simulink model "Punto1"  (R2017b)
settings: Solver=VariableStepAuto  StartTime=0.0  StopTime=5  RelTol=1e-3
values from neighbouring files (symbols this model uses):
  dc = [.4 4.2 3]    [Practica5.m]    (also in punto1.m)
  ddc = ddc(2:end)    [Practica5.m]    (also in punto1.m = [1 -0.8251 -0.1748])
  nc = 1    [Practica5.m]    (also in punto1.m)
  ndc = [dd]    [Practica5.m]    (also in punto1.m = [9.4518 -6.5019 0.0491])
  T0 = .5    (= 0.5)    [Practica5.m]    (also in punto1.m = 0.02)
settings Model: Creator=Agustin  LastModifiedBy=Agustin

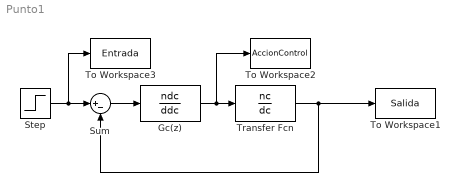
== system Punto1 ==
  Gc(z) : DiscreteTransferFcn  Numerator=ndc  Denominator=ddc  SampleTime=T0
  Step : Step  Time=0  SampleTime=T0
  Sum : Sum  Inputs=|+-
  To Workspace1 : ToWorkspace  VariableName=Salida  SaveFormat=Timeseries  SampleTime=-1
  To Workspace2 : ToWorkspace  VariableName=AccionControl  SaveFormat=Timeseries  SampleTime=-1
  To Workspace3 : ToWorkspace  VariableName=Entrada  SaveFormat=Timeseries  SampleTime=-1
  Transfer Fcn : TransferFcn  Numerator=nc  Denominator=dc
  wires:
  Transfer Fcn/1 -> To Workspace1/1, Sum/2
  Gc(z)/1 -> Transfer Fcn/1, To Workspace2/1
  Step/1 -> To Workspace3/1, Sum/1
  Sum/1 -> Gc(z)/1
